simulink model "dft"  (R2016b)
settings: Solver=VariableStepAuto  StartTime=0.0  StopTime=0.3  RelTol=1e-3
undefined symbols (not defined in the file or in its folder): get
libraries: dspspect3 x1, dspstat3 x1, dspsnks4 x1
settings Model: Creator=jeff  LastModifiedBy=jeff

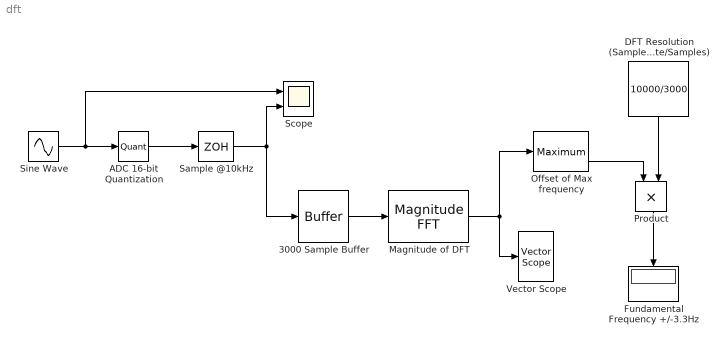
== system dft ==
  3000 Sample Buffer : Buffer  N=3000  TreatMby1Signals=One channel  OutputFrames=off
  ADC 16-bit Quantization : Quantizer  QuantizationInterval=1/ 2^15
  DFT Resolution (SampleRate/Samples) : Constant  Value=10000/3000
  Fundamental Frequency +/-3.3Hz : Display
  Magnitude of DFT : dspspect3/Magnitude FFT  mag_or_magsq=Magnitude squared  FFTImplementation=Auto  fftLenInherit=on  fftsize=256  WrapInput=on
  Offset of Max frequency : dspstat3/Maximum  operation=maximum  fcn=Value and Index  indexBase=One  operateOver=Each column  Dimension=1  InputProcessing=Columns as channels (frame based)  reset=None  roiEnable=off  roiType=Rectangles  roiPortion=Entire ROI  roiOutput=Individual statistics for each ROI  roiFlag=off  roundingMode=Floor  overflowMode=off  accumDataTypeStr=Inherit: Same as product output  accumLastDataTypeStr=Inherit: Same as product output
  Product : Product
  Sample @10kHz : ZeroOrderHold  SampleTime=1/10000
  Scope : Scope  NumInputPorts=2
  Sine Wave : Sin  Frequency=2*pi*1004  SampleTime=1/100000
  Vector Scope : dspsnks4/Vector Scope  ScopeProperties=on  Domain=Frequency  HorizSpan=1  DisplayProperties=off  AxisGrid=on  Memory=off  FrameNumber=on  AxisLegend=off  AxisZoom=off  OpenScopeAtSimStart=on  OpenScopeImmediately=off  FigPos=get(0,'defaultfigureposition')  AxisProperties=off  XUnits=Hertz  XRange=[0...Fs/2]  InheritXIncr=on  XIncr=1  XLabel=Time  XLimit=User-defined  XMin=0  XMax=5000  XStart=0  YUnits=dB  YLabel=Amplitude  LineProperties=off  LineMarkers=None  XAxisParamsVer=6.9
      settings: YMin=-6.3779  YMax=64.6308
  wires:
  Sine Wave/1 -> Scope/1, ADC 16-bit Quantization/1
  ADC 16-bit Quantization/1 -> Sample @10kHz/1
  Sample @10kHz/1 -> 3000 Sample Buffer/1, Scope/2
  Magnitude of DFT/1 -> Vector Scope/1, Offset of Max frequency/1
  3000 Sample Buffer/1 -> Magnitude of DFT/1
  Offset of Max frequency/2 -> Product/1
  Product/1 -> Fundamental Frequency +/-3.3Hz/1
  DFT Resolution (SampleRate/Samples)/1 -> Product/2
